simulink model "rc_circuit"  (R2020b)
settings: Solver=VariableStepAuto  StartTime=0.0  StopTime=10.0  RelTol=1e-3
model workspace (MAT data in the model file):
  C = Simulink.Parameter
  C.Value = 1e-05
  C.DataType = 'auto'
  C.Dimensions = [1 1]
  R = Simulink.Parameter
  R.Value = 10
  R.DataType = 'auto'
  R.Dimensions = [1 1]
settings Model: Creator=shivanshu shukla  LastModifiedBy=shivanshu shukla

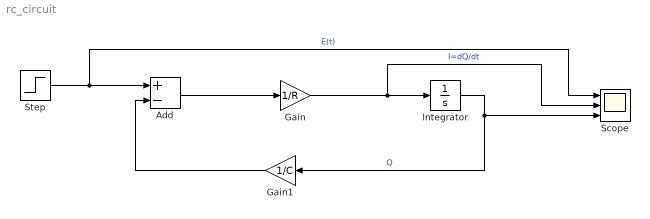
== system rc_circuit ==
  Add : Sum  Inputs=+-
  Gain : Gain  Gain=1/R
  Gain1 : Gain  Gain=1/C
  Integrator : Integrator  InitialCondition=1
  Scope : Scope  NumInputPorts=3
  Step : Step  After=5  SampleTime=0
  wires:
  Gain/1 -> Scope/2, Integrator/1  "I=dQ/dt"
  Add/1 -> Gain/1
  Integrator/1 -> Scope/3, Gain1/1  "Q"
  Gain1/1 -> Add/2
  Step/1 -> Scope/1, Add/1  "E(t)"
